simulink model "UAV3"  (R2024b)
settings: Solver=VariableStepAuto  StartTime=0.0  StopTime=tsim  RelTol=1e-3
values from neighbouring files (symbols this model uses):
  A = [ybb, yp+(w0/u0), yr-(u0/u0), g*cos(tt0)/u0 ... (first row only)    [init.m]    (also in new_A_B_integrativos.m = [A, zeros, zeros]; new_A_B_lambda.m = [A, zeros])
  B = [Yda, Ydr ... (first row only)    [init.m]    (also in new_A_B_integrativos.m = [B; new_line_bb; new_line_lambda]; new_A_B_lambda.m = [B; new_line_B])
  C = diag([1,1,1,1])    [main.m]    (also in untitled2.m)
  D = zeros(4,2)    [main.m]    (also in untitled2.m)
  u0 = u0*0.51444    (= 27.985536)    [Grupo3RP1.m]    (also in all_values.m; init.m = [da0, dr0]; untitled2.m)
  x0 = min(y_diff.signals.values)    [graficos_formacao.m]    (also in init.m = [0,0,0,0]; new_A_B_lambda.m = [0,0,0,0,0]')
settings Model: Creator=joaosantos  LastModifiedBy=ruben
settings DataIOCC: ReturnWorkspaceOutputs=off

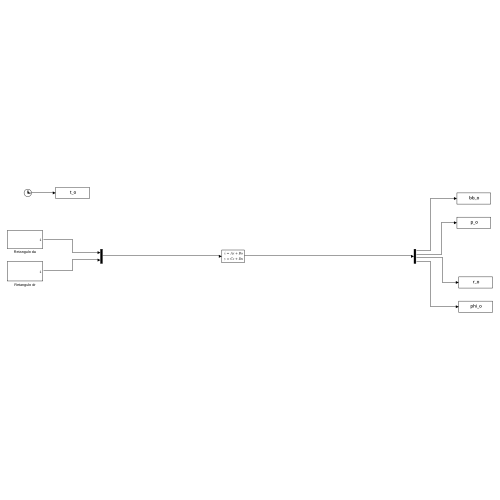
[thumbnail: Simulink's stored preview of the top-level diagram]
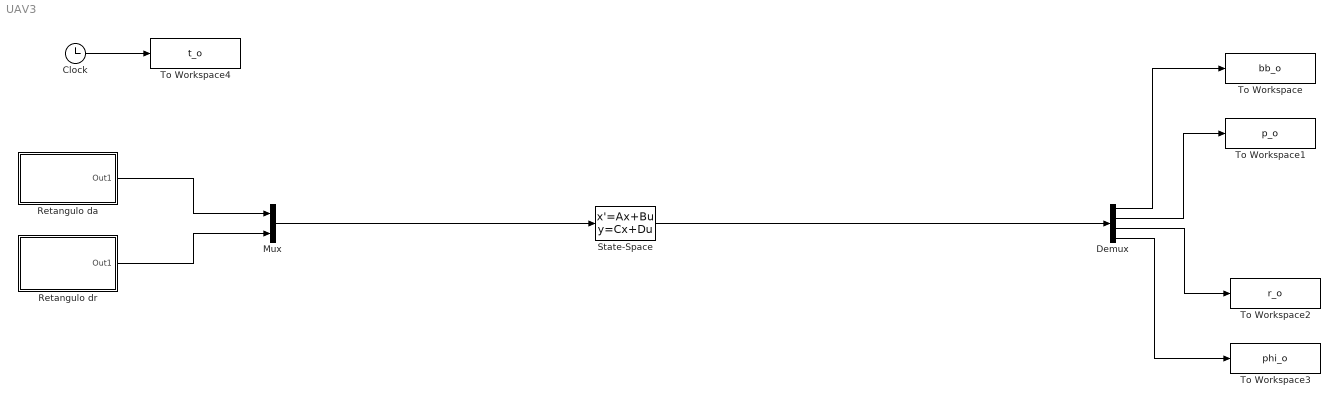
== system UAV3 ==
  Clock : Clock
  Demux : Demux
  Mux : Mux  Inputs=2
  Retangulo da : Subsystem
  Retangulo dr : Subsystem
  State-Space : StateSpace  A=A  B=B  C=C  D=D  InitialCondition=x0
  To Workspace : ToWorkspace  VariableName=bb_o  SampleTime=-1
  To Workspace1 : ToWorkspace  VariableName=p_o  SampleTime=-1
  To Workspace2 : ToWorkspace  VariableName=r_o  SampleTime=-1
  To Workspace3 : ToWorkspace  VariableName=phi_o  SampleTime=-1
  To Workspace4 : ToWorkspace  VariableName=t_o  SampleTime=-1
  wires:
  Demux/2 -> To Workspace1/1
  Demux/1 -> To Workspace/1
  Demux/3 -> To Workspace2/1
  Demux/4 -> To Workspace3/1
  Mux/1 -> State-Space/1
  State-Space/1 -> Demux/1
  Retangulo da/1(Out1) -> Mux/1
  Retangulo dr/1(Out1) -> Mux/2
  Clock/1 -> To Workspace4/1

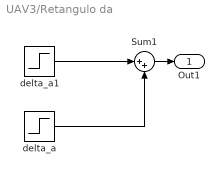
== system UAV3/Retangulo da ==
  Sum1 : Sum  Inputs=|++
  delta_a : Step  Time=10  After=u0(1)  SampleTime=0
  delta_a1 : Step  Time=25  After=-u0(1)  SampleTime=0
  Out1 : Outport
  wires:
  delta_a1/1 -> Sum1/1
  delta_a/1 -> Sum1/2
  Sum1/1 -> Out1/1

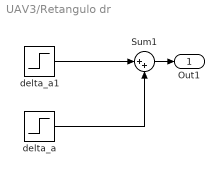
== system UAV3/Retangulo dr ==
  Sum1 : Sum  Inputs=|++
  delta_a : Step  Time=10  After=u0(2)  SampleTime=0
  delta_a1 : Step  Time=25  After=-u0(2)  SampleTime=0
  Out1 : Outport
  wires:
  delta_a1/1 -> Sum1/1
  delta_a/1 -> Sum1/2
  Sum1/1 -> Out1/1
